simulink model "mpcfinal"  (R2022a)
settings: Solver=VariableStepAuto  StartTime=0.0  StopTime=100  RelTol=1e-3
libraries: mpclib x5
settings Model: Creator=Admin  LastModifiedBy=Admin

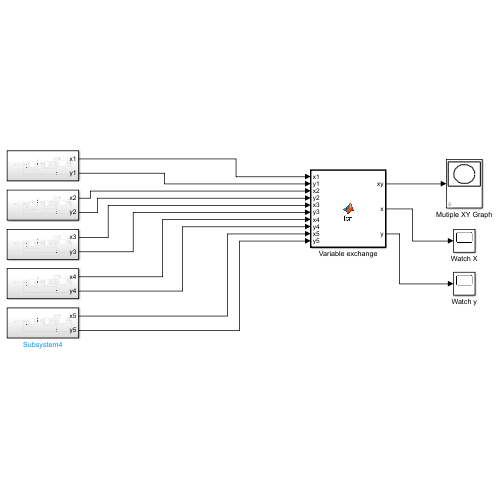
[thumbnail: Simulink's stored preview of the top-level diagram]
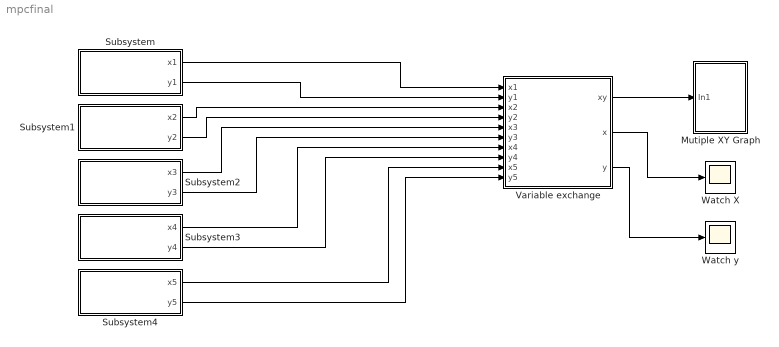
== system mpcfinal ==
  Mutiple XY Graph : Subsystem  mask(Mutiple XY Graph){number_of_trajectories=5, axis_limits=[-100 100 -100 100], sample_time=0.1}
      mask prompts: number_of_trajectories "Number of Trajectories"; axis_limits "Axis Limits"; sample_time "Sample Time"
      mask Display: plot([.05 .95 .95 .05 .05],[.45 .45 .95 .95 .45], 0.5+cos(0:0.1:2*pi)*0.3,0.7+sin(0:0.1:2*pi)*0.2)
  Subsystem : Subsystem
  Subsystem1 : Subsystem
  Subsystem2 : Subsystem
  Subsystem3 : Subsystem
  Subsystem4 : Subsystem
  Variable exchange : MATLAB Function  TreatAsAtomicUnit=on
  Watch X : Scope
  Watch y : Scope
  wires:
  Subsystem2/2(y3) -> Variable exchange/6(y3)
  Subsystem/2(y1) -> Variable exchange/2(y1)
  Subsystem4/2(y5) -> Variable exchange/10(y5)
  Subsystem2/1(x3) -> Variable exchange/5(x3)
  Subsystem4/1(x5) -> Variable exchange/9(x5)
  Variable exchange/1(xy) -> Mutiple XY Graph/1(In1)
  Variable exchange/2(x) -> Watch X/1
  Subsystem3/2(y4) -> Variable exchange/8(y4)
  Subsystem1/2(y2) -> Variable exchange/4(y2)
  Variable exchange/3(y) -> Watch y/1
  Subsystem1/1(x2) -> Variable exchange/3(x2)
  Subsystem/1(x1) -> Variable exchange/1(x1)
  Subsystem3/1(x4) -> Variable exchange/7(x4)

== system mpcfinal/Mutiple XY Graph ==
  In1 : Inport
  Level-2 MATLAB S-Function : M-S-Function  FunctionName=multiple_xy_graph  Parameters=number_of_trajectories,axis_limits
  Rate Transition : RateTransition  OutPortSampleTime=sample_time
  wires:
  In1/1 -> Rate Transition/1
  Rate Transition/1 -> Level-2 MATLAB S-Function/1

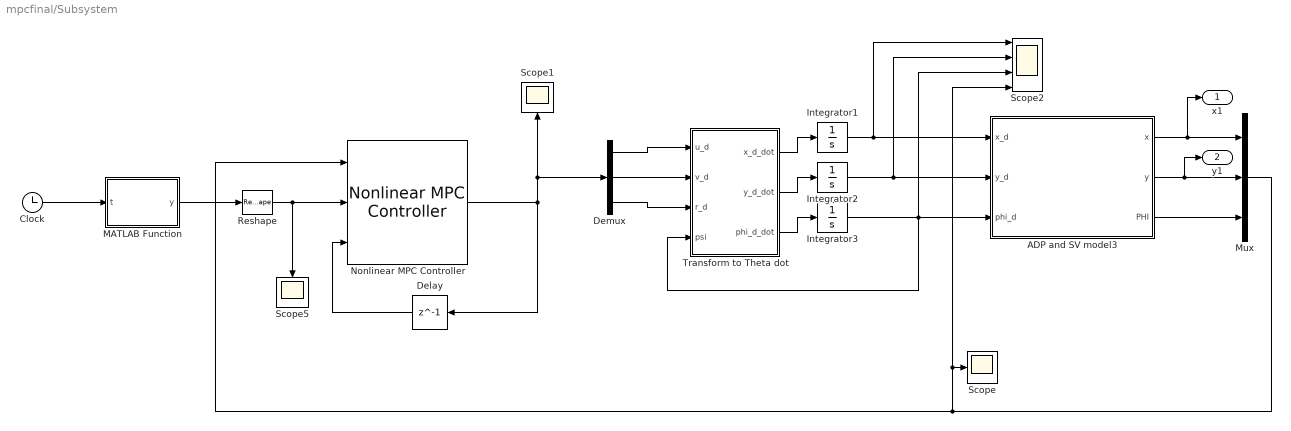
== system mpcfinal/Subsystem ==
  ADP and SV model3 : Subsystem
  Clock : Clock
  Delay : Delay  DelayLength=1
  Demux : Demux  Outputs=3
  Integrator1 : Integrator  InitialCondition=10
  Integrator2 : Integrator  InitialCondition=10
  Integrator3 : Integrator
  MATLAB Function : MATLAB Function  TreatAsAtomicUnit=on
  Mux : Mux  Inputs=3
  Nonlinear MPC Controller : mpclib/Nonlinear MPC Controller  nlmpcobj=nlobj  UseObjectTs=on  UseMEX=off  md_enabled=off  mvtarget_enabled=off  param_enabled=off  cost_enabled=off  mvseq_enabled=off  stateseq_enabled=off  ovseq_enabled=off  slack_enabled=off  status_enabled=off  ov_min=off  ov_max=off  mv_min=off  mv_max=off  mvrate_min=off  mvrate_max=off  state_min=off  state_max=off  ov_weight=off  mv_weight=off  mvrate_weight=off  ecr_weight=off  nlp_initialize=off
  Reshape : Reshape  OutputDimensionality=Customize  OutputDimensions=[1,3]
  Scope : Scope
  Scope1 : Scope
  Scope2 : Scope  NumInputPorts=4
  Scope5 : Scope
  Transform to Theta dot : MATLAB Function  TreatAsAtomicUnit=on
  x1 : Outport
  y1 : Outport  Port=2
  wires:
  Nonlinear MPC Controller/1 -> Demux/1, Scope1/1, Delay/1
  ADP and SV model3/2(y) -> y1/1, Mux/2
  ADP and SV model3/3(PHI) -> Mux/3
  Demux/1 -> Transform to Theta dot/1(u_d)
  Integrator2/1 -> ADP and SV model3/2(y_d), Scope2/2
  Clock/1 -> MATLAB Function/1(t)
  Transform to Theta dot/1(x_d_dot) -> Integrator1/1
  Reshape/1 -> Nonlinear MPC Controller/2, Scope5/1
  Integrator3/1 -> ADP and SV model3/3(phi_d), Transform to Theta dot/4(psi), Scope2/3
  MATLAB Function/1(y) -> Reshape/1
  Demux/3 -> Transform to Theta dot/3(r_d)
  ADP and SV model3/1(x) -> x1/1, Mux/1
  Delay/1 -> Nonlinear MPC Controller/3
  Transform to Theta dot/2(y_d_dot) -> Integrator2/1
  Demux/2 -> Transform to Theta dot/2(v_d)
  Mux/1 -> Scope2/4, Scope/1, Nonlinear MPC Controller/1
  Integrator1/1 -> Scope2/1, ADP and SV model3/1(x_d)
  Transform to Theta dot/3(phi_d_dot) -> Integrator3/1

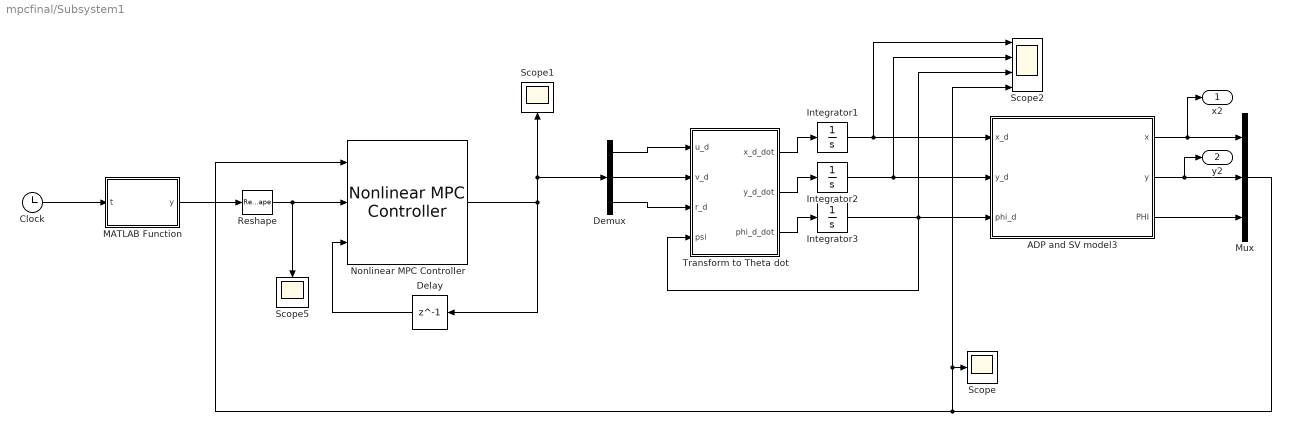
== system mpcfinal/Subsystem1 ==
  ADP and SV model3 : Subsystem
  Clock : Clock
  Delay : Delay  DelayLength=1
  Demux : Demux  Outputs=3
  Integrator1 : Integrator  InitialCondition=15
  Integrator2 : Integrator  InitialCondition=10
  Integrator3 : Integrator
  MATLAB Function : MATLAB Function  TreatAsAtomicUnit=on
  Mux : Mux  Inputs=3
  Nonlinear MPC Controller : mpclib/Nonlinear MPC Controller  nlmpcobj=nlobj  UseObjectTs=on  UseMEX=off  md_enabled=off  mvtarget_enabled=off  param_enabled=off  cost_enabled=off  mvseq_enabled=off  stateseq_enabled=off  ovseq_enabled=off  slack_enabled=off  status_enabled=off  ov_min=off  ov_max=off  mv_min=off  mv_max=off  mvrate_min=off  mvrate_max=off  state_min=off  state_max=off  ov_weight=off  mv_weight=off  mvrate_weight=off  ecr_weight=off  nlp_initialize=off
  Reshape : Reshape  OutputDimensionality=Customize  OutputDimensions=[1,3]
  Scope : Scope
  Scope1 : Scope
  Scope2 : Scope  NumInputPorts=4
  Scope5 : Scope
  Transform to Theta dot : MATLAB Function  TreatAsAtomicUnit=on
  x2 : Outport
  y2 : Outport  Port=2
  wires:
  Nonlinear MPC Controller/1 -> Demux/1, Scope1/1, Delay/1
  ADP and SV model3/2(y) -> y2/1, Mux/2
  ADP and SV model3/3(PHI) -> Mux/3
  Demux/1 -> Transform to Theta dot/1(u_d)
  Integrator2/1 -> ADP and SV model3/2(y_d), Scope2/2
  Clock/1 -> MATLAB Function/1(t)
  Transform to Theta dot/1(x_d_dot) -> Integrator1/1
  Reshape/1 -> Nonlinear MPC Controller/2, Scope5/1
  Integrator3/1 -> ADP and SV model3/3(phi_d), Transform to Theta dot/4(psi), Scope2/3
  MATLAB Function/1(y) -> Reshape/1
  Demux/3 -> Transform to Theta dot/3(r_d)
  ADP and SV model3/1(x) -> x2/1, Mux/1
  Delay/1 -> Nonlinear MPC Controller/3
  Transform to Theta dot/2(y_d_dot) -> Integrator2/1
  Demux/2 -> Transform to Theta dot/2(v_d)
  Mux/1 -> Scope2/4, Scope/1, Nonlinear MPC Controller/1
  Integrator1/1 -> Scope2/1, ADP and SV model3/1(x_d)
  Transform to Theta dot/3(phi_d_dot) -> Integrator3/1

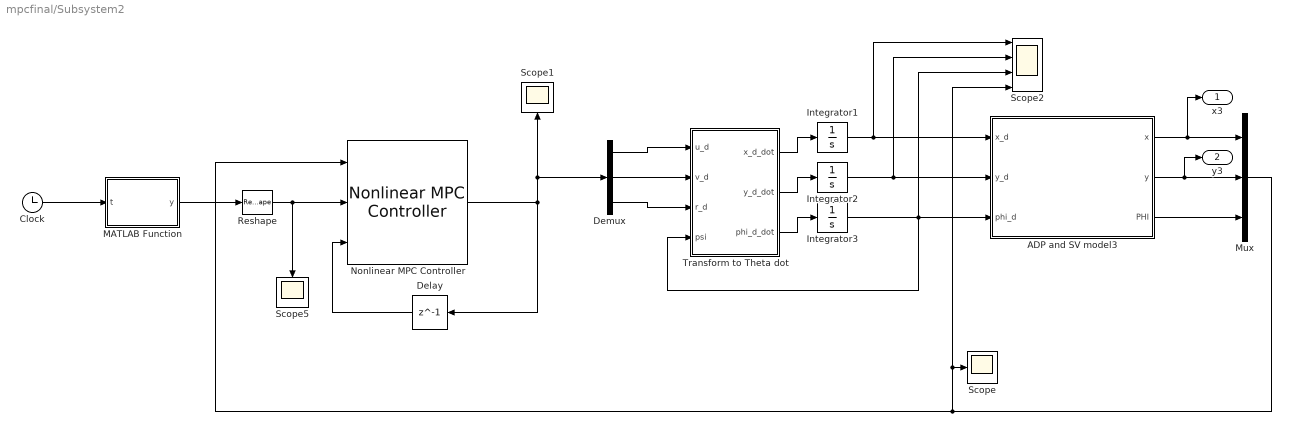
== system mpcfinal/Subsystem2 ==
  ADP and SV model3 : Subsystem
  Clock : Clock
  Delay : Delay  DelayLength=1
  Demux : Demux  Outputs=3
  Integrator1 : Integrator  InitialCondition=10
  Integrator2 : Integrator  InitialCondition=5
  Integrator3 : Integrator
  MATLAB Function : MATLAB Function  TreatAsAtomicUnit=on
  Mux : Mux  Inputs=3
  Nonlinear MPC Controller : mpclib/Nonlinear MPC Controller  nlmpcobj=nlobj  UseObjectTs=on  UseMEX=off  md_enabled=off  mvtarget_enabled=off  param_enabled=off  cost_enabled=off  mvseq_enabled=off  stateseq_enabled=off  ovseq_enabled=off  slack_enabled=off  status_enabled=off  ov_min=off  ov_max=off  mv_min=off  mv_max=off  mvrate_min=off  mvrate_max=off  state_min=off  state_max=off  ov_weight=off  mv_weight=off  mvrate_weight=off  ecr_weight=off  nlp_initialize=off
  Reshape : Reshape  OutputDimensionality=Customize  OutputDimensions=[1,3]
  Scope : Scope
  Scope1 : Scope
  Scope2 : Scope  NumInputPorts=4
  Scope5 : Scope
  Transform to Theta dot : MATLAB Function  TreatAsAtomicUnit=on
  x3 : Outport
  y3 : Outport  Port=2
  wires:
  Nonlinear MPC Controller/1 -> Demux/1, Scope1/1, Delay/1
  ADP and SV model3/2(y) -> y3/1, Mux/2
  ADP and SV model3/3(PHI) -> Mux/3
  Demux/1 -> Transform to Theta dot/1(u_d)
  Integrator2/1 -> ADP and SV model3/2(y_d), Scope2/2
  Clock/1 -> MATLAB Function/1(t)
  Transform to Theta dot/1(x_d_dot) -> Integrator1/1
  Reshape/1 -> Nonlinear MPC Controller/2, Scope5/1
  Integrator3/1 -> ADP and SV model3/3(phi_d), Transform to Theta dot/4(psi), Scope2/3
  MATLAB Function/1(y) -> Reshape/1
  Demux/3 -> Transform to Theta dot/3(r_d)
  ADP and SV model3/1(x) -> x3/1, Mux/1
  Delay/1 -> Nonlinear MPC Controller/3
  Transform to Theta dot/2(y_d_dot) -> Integrator2/1
  Demux/2 -> Transform to Theta dot/2(v_d)
  Mux/1 -> Scope2/4, Scope/1, Nonlinear MPC Controller/1
  Integrator1/1 -> Scope2/1, ADP and SV model3/1(x_d)
  Transform to Theta dot/3(phi_d_dot) -> Integrator3/1

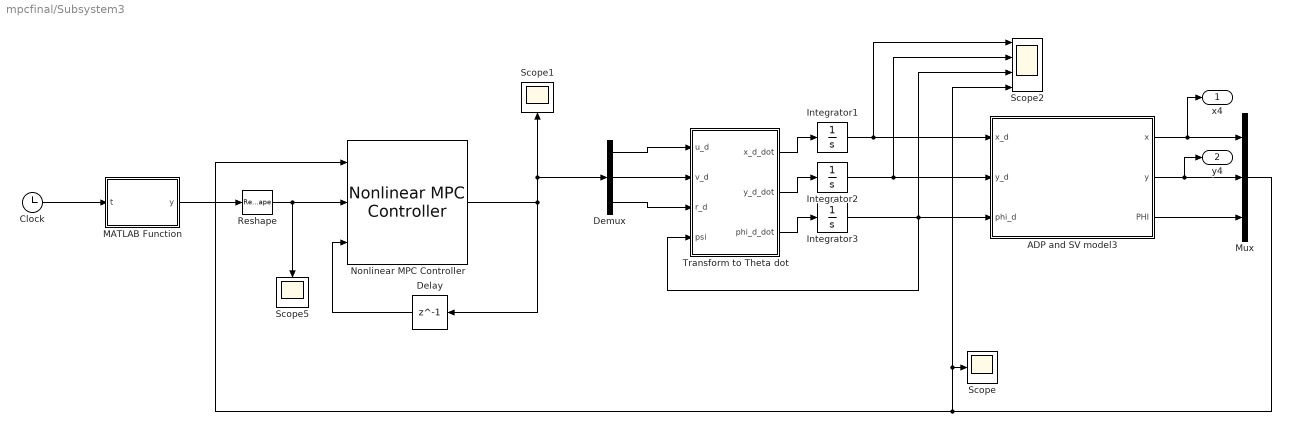
== system mpcfinal/Subsystem3 ==
  ADP and SV model3 : Subsystem
  Clock : Clock
  Delay : Delay  DelayLength=1
  Demux : Demux  Outputs=3
  Integrator1 : Integrator  InitialCondition=5
  Integrator2 : Integrator  InitialCondition=10
  Integrator3 : Integrator
  MATLAB Function : MATLAB Function  TreatAsAtomicUnit=on
  Mux : Mux  Inputs=3
  Nonlinear MPC Controller : mpclib/Nonlinear MPC Controller  nlmpcobj=nlobj  UseObjectTs=on  UseMEX=off  md_enabled=off  mvtarget_enabled=off  param_enabled=off  cost_enabled=off  mvseq_enabled=off  stateseq_enabled=off  ovseq_enabled=off  slack_enabled=off  status_enabled=off  ov_min=off  ov_max=off  mv_min=off  mv_max=off  mvrate_min=off  mvrate_max=off  state_min=off  state_max=off  ov_weight=off  mv_weight=off  mvrate_weight=off  ecr_weight=off  nlp_initialize=off
  Reshape : Reshape  OutputDimensionality=Customize  OutputDimensions=[1,3]
  Scope : Scope
  Scope1 : Scope
  Scope2 : Scope  NumInputPorts=4
  Scope5 : Scope
  Transform to Theta dot : MATLAB Function  TreatAsAtomicUnit=on
  x4 : Outport
  y4 : Outport  Port=2
  wires:
  Nonlinear MPC Controller/1 -> Demux/1, Scope1/1, Delay/1
  ADP and SV model3/2(y) -> y4/1, Mux/2
  ADP and SV model3/3(PHI) -> Mux/3
  Demux/1 -> Transform to Theta dot/1(u_d)
  Integrator2/1 -> ADP and SV model3/2(y_d), Scope2/2
  Clock/1 -> MATLAB Function/1(t)
  Transform to Theta dot/1(x_d_dot) -> Integrator1/1
  Reshape/1 -> Nonlinear MPC Controller/2, Scope5/1
  Integrator3/1 -> ADP and SV model3/3(phi_d), Transform to Theta dot/4(psi), Scope2/3
  MATLAB Function/1(y) -> Reshape/1
  Demux/3 -> Transform to Theta dot/3(r_d)
  ADP and SV model3/1(x) -> x4/1, Mux/1
  Delay/1 -> Nonlinear MPC Controller/3
  Transform to Theta dot/2(y_d_dot) -> Integrator2/1
  Demux/2 -> Transform to Theta dot/2(v_d)
  Mux/1 -> Scope2/4, Scope/1, Nonlinear MPC Controller/1
  Integrator1/1 -> Scope2/1, ADP and SV model3/1(x_d)
  Transform to Theta dot/3(phi_d_dot) -> Integrator3/1

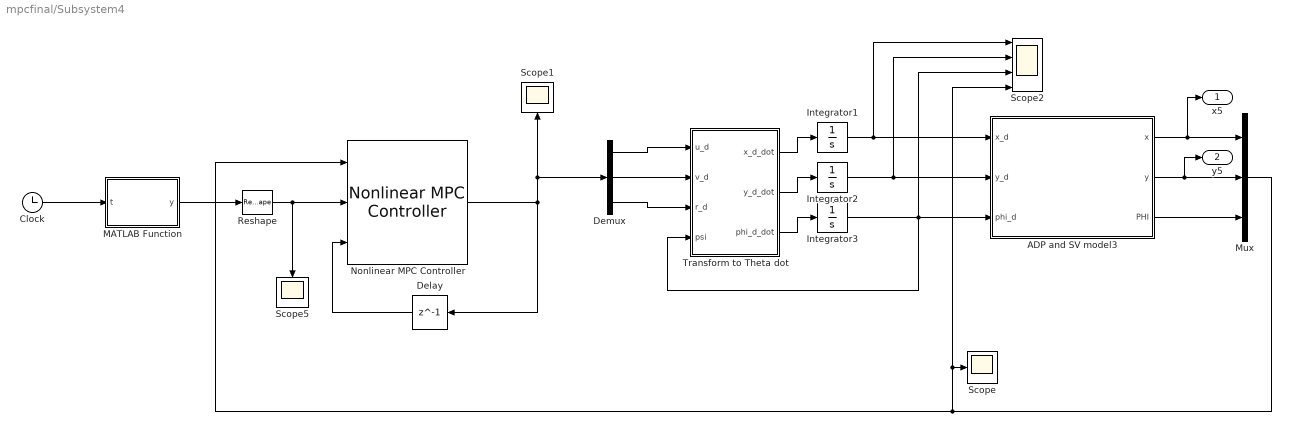
== system mpcfinal/Subsystem4 ==
  ADP and SV model3 : Subsystem
  Clock : Clock
  Delay : Delay  DelayLength=1
  Demux : Demux  Outputs=3
  Integrator1 : Integrator  InitialCondition=10
  Integrator2 : Integrator  InitialCondition=15
  Integrator3 : Integrator
  MATLAB Function : MATLAB Function  TreatAsAtomicUnit=on
  Mux : Mux  Inputs=3
  Nonlinear MPC Controller : mpclib/Nonlinear MPC Controller  nlmpcobj=nlobj  UseObjectTs=on  UseMEX=off  md_enabled=off  mvtarget_enabled=off  param_enabled=off  cost_enabled=off  mvseq_enabled=off  stateseq_enabled=off  ovseq_enabled=off  slack_enabled=off  status_enabled=off  ov_min=off  ov_max=off  mv_min=off  mv_max=off  mvrate_min=off  mvrate_max=off  state_min=off  state_max=off  ov_weight=off  mv_weight=off  mvrate_weight=off  ecr_weight=off  nlp_initialize=off
  Reshape : Reshape  OutputDimensionality=Customize  OutputDimensions=[1,3]
  Scope : Scope
  Scope1 : Scope
  Scope2 : Scope  NumInputPorts=4
  Scope5 : Scope
  Transform to Theta dot : MATLAB Function  TreatAsAtomicUnit=on
  x5 : Outport
  y5 : Outport  Port=2
  wires:
  Nonlinear MPC Controller/1 -> Demux/1, Scope1/1, Delay/1
  ADP and SV model3/2(y) -> y5/1, Mux/2
  ADP and SV model3/3(PHI) -> Mux/3
  Demux/1 -> Transform to Theta dot/1(u_d)
  Integrator2/1 -> ADP and SV model3/2(y_d), Scope2/2
  Clock/1 -> MATLAB Function/1(t)
  Transform to Theta dot/1(x_d_dot) -> Integrator1/1
  Reshape/1 -> Nonlinear MPC Controller/2, Scope5/1
  Integrator3/1 -> ADP and SV model3/3(phi_d), Transform to Theta dot/4(psi), Scope2/3
  MATLAB Function/1(y) -> Reshape/1
  Demux/3 -> Transform to Theta dot/3(r_d)
  ADP and SV model3/1(x) -> x5/1, Mux/1
  Delay/1 -> Nonlinear MPC Controller/3
  Transform to Theta dot/2(y_d_dot) -> Integrator2/1
  Demux/2 -> Transform to Theta dot/2(v_d)
  Mux/1 -> Scope2/4, Scope/1, Nonlinear MPC Controller/1
  Integrator1/1 -> Scope2/1, ADP and SV model3/1(x_d)
  Transform to Theta dot/3(phi_d_dot) -> Integrator3/1

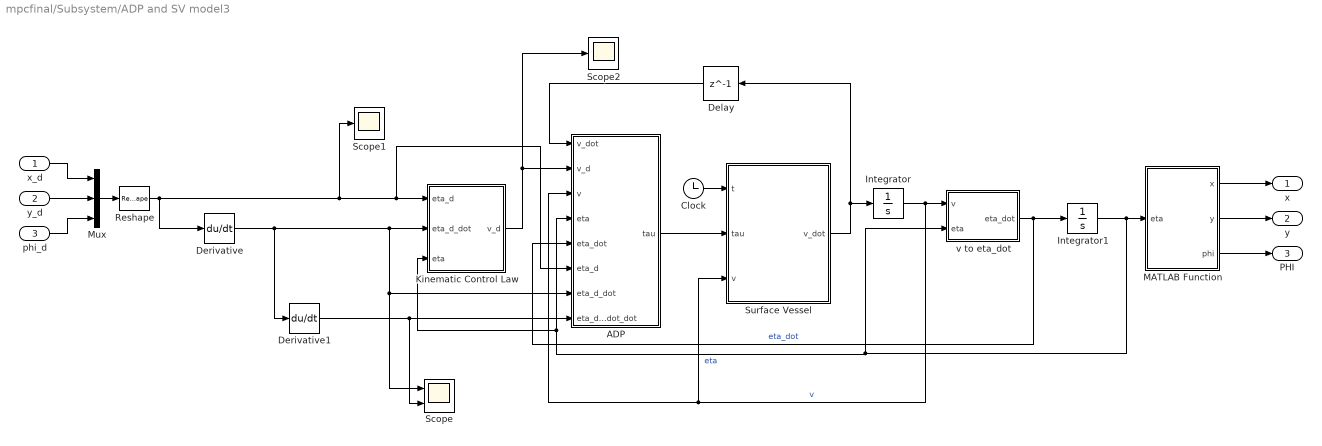
== system mpcfinal/Subsystem/ADP and SV model3 ==
  x_d : Inport
  y_d : Inport  Port=2
  phi_d : Inport  Port=3
  ADP : Subsystem
  Clock : Clock
  Delay : Delay  DelayLength=1  InitialCondition=[0;0;0]  SampleTime=1e-2
  Derivative : Derivative
  Derivative1 : Derivative
  Integrator : Integrator
  Integrator1 : Integrator  InitialCondition=[9;11;0.1]
  "Kinematic Control Law " : MATLAB Function  TreatAsAtomicUnit=on
  MATLAB Function : MATLAB Function  TreatAsAtomicUnit=on
  Mux : Mux  Inputs=3
  Reshape : Reshape  OutputDimensionality=Customize  OutputDimensions=[3,1]
  Scope : Scope  NumInputPorts=2
  Scope1 : Scope
  Scope2 : Scope
  "Surface Vessel " : MATLAB Function  TreatAsAtomicUnit=on
  v to eta_dot : MATLAB Function  TreatAsAtomicUnit=on
  x : Outport
  y : Outport  Port=2
  PHI : Outport  Port=3
  wires:
  x_d/1 -> Mux/1
  phi_d/1 -> Mux/3
  y_d/1 -> Mux/2
  Clock/1 -> "Surface Vessel "/1(t)
  "Surface Vessel "/1(v_dot) -> Delay/1, Integrator/1
  Integrator/1 -> ADP/3(v), "Surface Vessel "/3(v), v to eta_dot/1(v)  "v"
  Integrator1/1 -> ADP/4(eta), "Kinematic Control Law "/3(eta), v to eta_dot/2(eta), MATLAB Function/1(eta)  "eta"
  ADP/1(tau) -> "Surface Vessel "/2(tau)
  "Kinematic Control Law "/1(v_d) -> Scope2/1, ADP/2(v_d)
  Delay/1 -> ADP/1(v_dot)
  Reshape/1 -> Derivative/1, Scope1/1, ADP/6(eta_d), "Kinematic Control Law "/1(eta_d)
  v to eta_dot/1(eta_dot) -> ADP/5(eta_dot), Integrator1/1  "eta_dot"
  MATLAB Function/1(x) -> x/1
  MATLAB Function/2(y) -> y/1
  MATLAB Function/3(phi) -> PHI/1
  Mux/1 -> Reshape/1
  Derivative/1 -> Derivative1/1, ADP/7(eta_d_dot), Scope/1, "Kinematic Control Law "/2(eta_d_dot)
  Derivative1/1 -> Scope/2, ADP/8(eta_d_dot_dot)

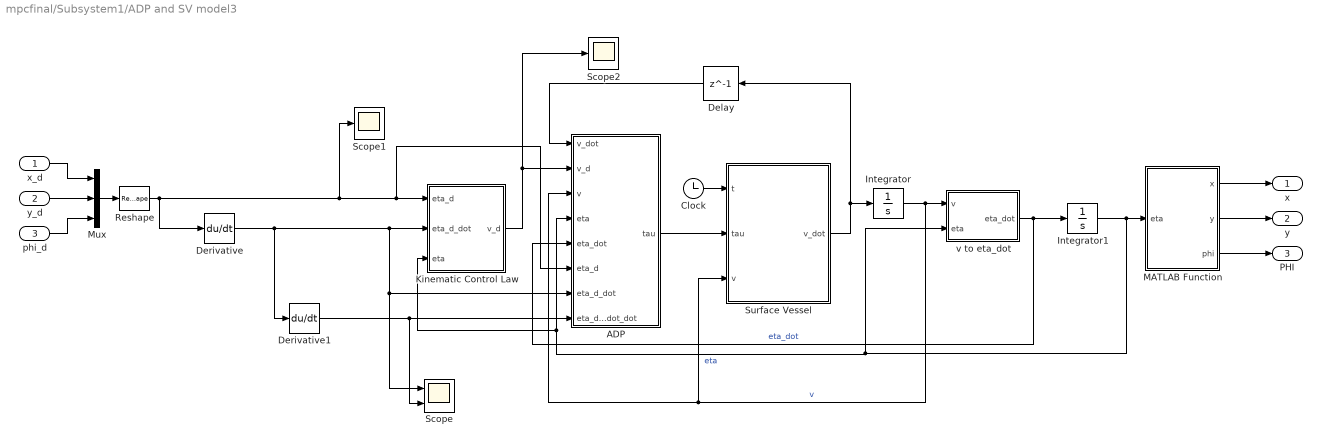
== system mpcfinal/Subsystem1/ADP and SV model3 ==
  x_d : Inport
  y_d : Inport  Port=2
  phi_d : Inport  Port=3
  ADP : Subsystem
  Clock : Clock
  Delay : Delay  DelayLength=1  InitialCondition=[0;0;0]  SampleTime=1e-2
  Derivative : Derivative
  Derivative1 : Derivative
  Integrator : Integrator
  Integrator1 : Integrator  InitialCondition=[14;11;0.1]
  "Kinematic Control Law " : MATLAB Function  TreatAsAtomicUnit=on
  MATLAB Function : MATLAB Function  TreatAsAtomicUnit=on
  Mux : Mux  Inputs=3
  Reshape : Reshape  OutputDimensionality=Customize  OutputDimensions=[3,1]
  Scope : Scope  NumInputPorts=2
  Scope1 : Scope
  Scope2 : Scope
  "Surface Vessel " : MATLAB Function  TreatAsAtomicUnit=on
  v to eta_dot : MATLAB Function  TreatAsAtomicUnit=on
  x : Outport
  y : Outport  Port=2
  PHI : Outport  Port=3
  wires:
  x_d/1 -> Mux/1
  phi_d/1 -> Mux/3
  y_d/1 -> Mux/2
  Clock/1 -> "Surface Vessel "/1(t)
  "Surface Vessel "/1(v_dot) -> Delay/1, Integrator/1
  Integrator/1 -> ADP/3(v), "Surface Vessel "/3(v), v to eta_dot/1(v)  "v"
  Integrator1/1 -> ADP/4(eta), "Kinematic Control Law "/3(eta), v to eta_dot/2(eta), MATLAB Function/1(eta)  "eta"
  ADP/1(tau) -> "Surface Vessel "/2(tau)
  "Kinematic Control Law "/1(v_d) -> Scope2/1, ADP/2(v_d)
  Delay/1 -> ADP/1(v_dot)
  Reshape/1 -> Derivative/1, Scope1/1, ADP/6(eta_d), "Kinematic Control Law "/1(eta_d)
  v to eta_dot/1(eta_dot) -> ADP/5(eta_dot), Integrator1/1  "eta_dot"
  MATLAB Function/1(x) -> x/1
  MATLAB Function/2(y) -> y/1
  MATLAB Function/3(phi) -> PHI/1
  Mux/1 -> Reshape/1
  Derivative/1 -> Derivative1/1, ADP/7(eta_d_dot), Scope/1, "Kinematic Control Law "/2(eta_d_dot)
  Derivative1/1 -> Scope/2, ADP/8(eta_d_dot_dot)

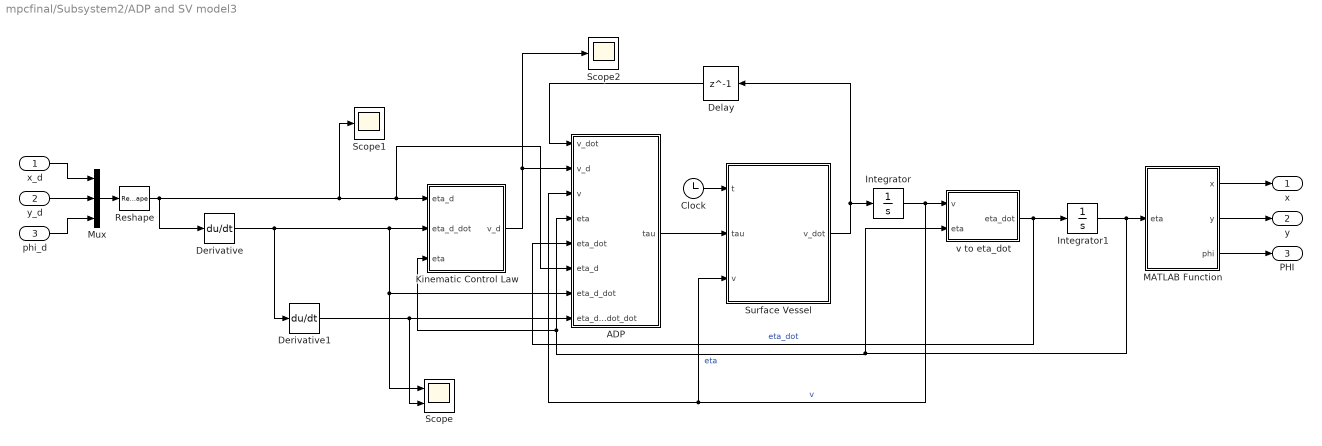
== system mpcfinal/Subsystem2/ADP and SV model3 ==
  x_d : Inport
  y_d : Inport  Port=2
  phi_d : Inport  Port=3
  ADP : Subsystem
  Clock : Clock
  Delay : Delay  DelayLength=1  InitialCondition=[0;0;0]  SampleTime=1e-2
  Derivative : Derivative
  Derivative1 : Derivative
  Integrator : Integrator
  Integrator1 : Integrator  InitialCondition=[9;5;-0.1]
  "Kinematic Control Law " : MATLAB Function  TreatAsAtomicUnit=on
  MATLAB Function : MATLAB Function  TreatAsAtomicUnit=on
  Mux : Mux  Inputs=3
  Reshape : Reshape  OutputDimensionality=Customize  OutputDimensions=[3,1]
  Scope : Scope  NumInputPorts=2
  Scope1 : Scope
  Scope2 : Scope
  "Surface Vessel " : MATLAB Function  TreatAsAtomicUnit=on
  v to eta_dot : MATLAB Function  TreatAsAtomicUnit=on
  x : Outport
  y : Outport  Port=2
  PHI : Outport  Port=3
  wires:
  x_d/1 -> Mux/1
  phi_d/1 -> Mux/3
  y_d/1 -> Mux/2
  Clock/1 -> "Surface Vessel "/1(t)
  "Surface Vessel "/1(v_dot) -> Delay/1, Integrator/1
  Integrator/1 -> ADP/3(v), "Surface Vessel "/3(v), v to eta_dot/1(v)  "v"
  Integrator1/1 -> ADP/4(eta), "Kinematic Control Law "/3(eta), v to eta_dot/2(eta), MATLAB Function/1(eta)  "eta"
  ADP/1(tau) -> "Surface Vessel "/2(tau)
  "Kinematic Control Law "/1(v_d) -> Scope2/1, ADP/2(v_d)
  Delay/1 -> ADP/1(v_dot)
  Reshape/1 -> Derivative/1, Scope1/1, ADP/6(eta_d), "Kinematic Control Law "/1(eta_d)
  v to eta_dot/1(eta_dot) -> ADP/5(eta_dot), Integrator1/1  "eta_dot"
  MATLAB Function/1(x) -> x/1
  MATLAB Function/2(y) -> y/1
  MATLAB Function/3(phi) -> PHI/1
  Mux/1 -> Reshape/1
  Derivative/1 -> Derivative1/1, ADP/7(eta_d_dot), Scope/1, "Kinematic Control Law "/2(eta_d_dot)
  Derivative1/1 -> Scope/2, ADP/8(eta_d_dot_dot)

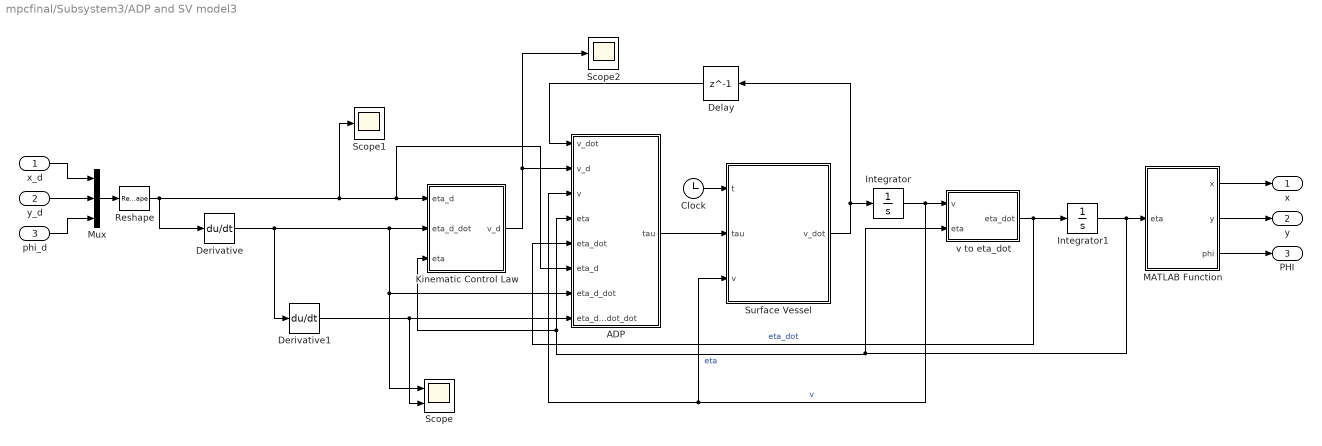
== system mpcfinal/Subsystem3/ADP and SV model3 ==
  x_d : Inport
  y_d : Inport  Port=2
  phi_d : Inport  Port=3
  ADP : Subsystem
  Clock : Clock
  Delay : Delay  DelayLength=1  InitialCondition=[0;0;0]  SampleTime=1e-2
  Derivative : Derivative
  Derivative1 : Derivative
  Integrator : Integrator
  Integrator1 : Integrator  InitialCondition=[6;11;0.1]
  "Kinematic Control Law " : MATLAB Function  TreatAsAtomicUnit=on
  MATLAB Function : MATLAB Function  TreatAsAtomicUnit=on
  Mux : Mux  Inputs=3
  Reshape : Reshape  OutputDimensionality=Customize  OutputDimensions=[3,1]
  Scope : Scope  NumInputPorts=2
  Scope1 : Scope
  Scope2 : Scope
  "Surface Vessel " : MATLAB Function  TreatAsAtomicUnit=on
  v to eta_dot : MATLAB Function  TreatAsAtomicUnit=on
  x : Outport
  y : Outport  Port=2
  PHI : Outport  Port=3
  wires:
  x_d/1 -> Mux/1
  phi_d/1 -> Mux/3
  y_d/1 -> Mux/2
  Clock/1 -> "Surface Vessel "/1(t)
  "Surface Vessel "/1(v_dot) -> Delay/1, Integrator/1
  Integrator/1 -> ADP/3(v), "Surface Vessel "/3(v), v to eta_dot/1(v)  "v"
  Integrator1/1 -> ADP/4(eta), "Kinematic Control Law "/3(eta), v to eta_dot/2(eta), MATLAB Function/1(eta)  "eta"
  ADP/1(tau) -> "Surface Vessel "/2(tau)
  "Kinematic Control Law "/1(v_d) -> Scope2/1, ADP/2(v_d)
  Delay/1 -> ADP/1(v_dot)
  Reshape/1 -> Derivative/1, Scope1/1, ADP/6(eta_d), "Kinematic Control Law "/1(eta_d)
  v to eta_dot/1(eta_dot) -> ADP/5(eta_dot), Integrator1/1  "eta_dot"
  MATLAB Function/1(x) -> x/1
  MATLAB Function/2(y) -> y/1
  MATLAB Function/3(phi) -> PHI/1
  Mux/1 -> Reshape/1
  Derivative/1 -> Derivative1/1, ADP/7(eta_d_dot), Scope/1, "Kinematic Control Law "/2(eta_d_dot)
  Derivative1/1 -> Scope/2, ADP/8(eta_d_dot_dot)

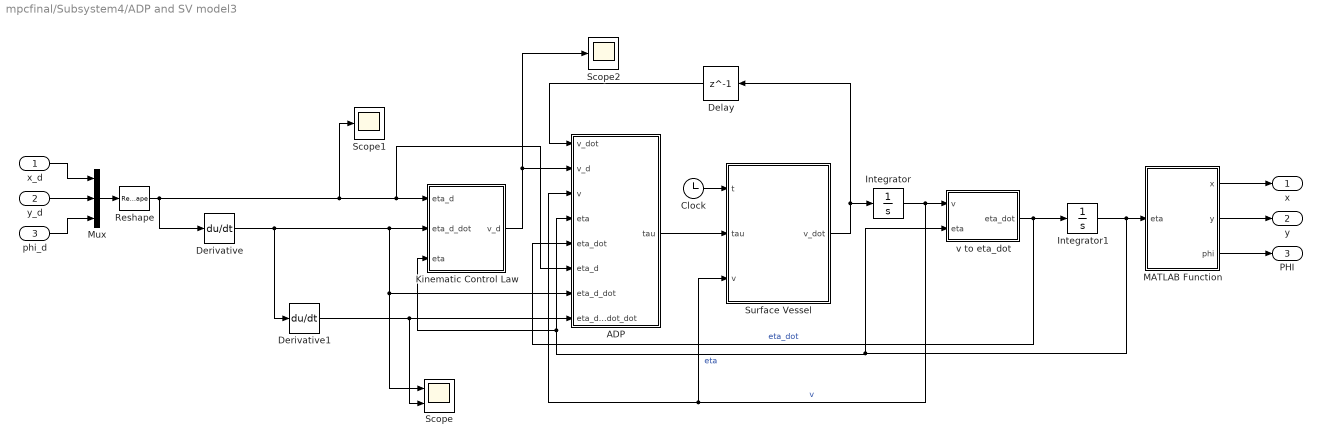
== system mpcfinal/Subsystem4/ADP and SV model3 ==
  x_d : Inport
  y_d : Inport  Port=2
  phi_d : Inport  Port=3
  ADP : Subsystem
  Clock : Clock
  Delay : Delay  DelayLength=1  InitialCondition=[0;0;0]  SampleTime=1e-2
  Derivative : Derivative
  Derivative1 : Derivative
  Integrator : Integrator
  Integrator1 : Integrator  InitialCondition=[9;14;-0.1]
  "Kinematic Control Law " : MATLAB Function  TreatAsAtomicUnit=on
  MATLAB Function : MATLAB Function  TreatAsAtomicUnit=on
  Mux : Mux  Inputs=3
  Reshape : Reshape  OutputDimensionality=Customize  OutputDimensions=[3,1]
  Scope : Scope  NumInputPorts=2
  Scope1 : Scope
  Scope2 : Scope
  "Surface Vessel " : MATLAB Function  TreatAsAtomicUnit=on
  v to eta_dot : MATLAB Function  TreatAsAtomicUnit=on
  x : Outport
  y : Outport  Port=2
  PHI : Outport  Port=3
  wires:
  x_d/1 -> Mux/1
  phi_d/1 -> Mux/3
  y_d/1 -> Mux/2
  Clock/1 -> "Surface Vessel "/1(t)
  "Surface Vessel "/1(v_dot) -> Delay/1, Integrator/1
  Integrator/1 -> ADP/3(v), "Surface Vessel "/3(v), v to eta_dot/1(v)  "v"
  Integrator1/1 -> ADP/4(eta), "Kinematic Control Law "/3(eta), v to eta_dot/2(eta), MATLAB Function/1(eta)  "eta"
  ADP/1(tau) -> "Surface Vessel "/2(tau)
  "Kinematic Control Law "/1(v_d) -> Scope2/1, ADP/2(v_d)
  Delay/1 -> ADP/1(v_dot)
  Reshape/1 -> Derivative/1, Scope1/1, ADP/6(eta_d), "Kinematic Control Law "/1(eta_d)
  v to eta_dot/1(eta_dot) -> ADP/5(eta_dot), Integrator1/1  "eta_dot"
  MATLAB Function/1(x) -> x/1
  MATLAB Function/2(y) -> y/1
  MATLAB Function/3(phi) -> PHI/1
  Mux/1 -> Reshape/1
  Derivative/1 -> Derivative1/1, ADP/7(eta_d_dot), Scope/1, "Kinematic Control Law "/2(eta_d_dot)
  Derivative1/1 -> Scope/2, ADP/8(eta_d_dot_dot)

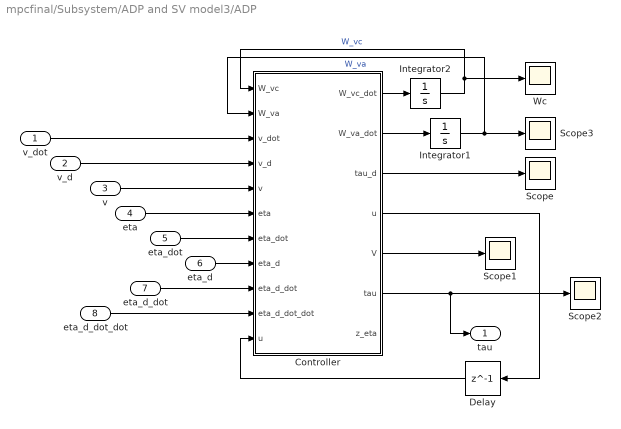
== system mpcfinal/Subsystem/ADP and SV model3/ADP ==
  v_dot : Inport
  v_d : Inport  Port=2
  v : Inport  Port=3
  eta : Inport  Port=4
  eta_dot : Inport  Port=5
  eta_d : Inport  Port=6
  eta_d_dot : Inport  Port=7
  eta_d_dot_dot : Inport  Port=8
  Controller : MATLAB Function  TreatAsAtomicUnit=on
  Delay : Delay  DelayLength=1  InitialCondition=[0;0;0]  SampleTime=1e-2
  Integrator1 : Integrator  InitialCondition=zeros(12,1)+0.1
  Integrator2 : Integrator  InitialCondition=zeros(12,1)
  Scope{,1..3} (4 alike) : Scope
  Wc : Scope
  tau : Outport
  wires:
  Controller/1(W_vc_dot) -> Integrator2/1
  Controller/2(W_va_dot) -> Integrator1/1
  Integrator1/1 -> Scope3/1, Controller/2(W_va)  "W_va"
  Integrator2/1 -> Controller/1(W_vc), Wc/1  "W_vc"
  v_d/1 -> Controller/4(v_d)
  v/1 -> Controller/5(v)
  eta/1 -> Controller/6(eta)
  eta_d/1 -> Controller/8(eta_d)
  eta_d_dot/1 -> Controller/9(eta_d_dot)
  eta_d_dot_dot/1 -> Controller/10(eta_d_dot_dot)
  eta_dot/1 -> Controller/7(eta_dot)
  Delay/1 -> Controller/11("u ")
  v_dot/1 -> Controller/3(v_dot)
  Controller/4(u) -> Delay/1
  Controller/6(tau) -> tau/1, Scope2/1
  Controller/3(tau_d) -> Scope/1
  Controller/5(V) -> Scope1/1

== system mpcfinal/Subsystem1/ADP and SV model3/ADP ==
  v_dot : Inport
  v_d : Inport  Port=2
  v : Inport  Port=3
  eta : Inport  Port=4
  eta_dot : Inport  Port=5
  eta_d : Inport  Port=6
  eta_d_dot : Inport  Port=7
  eta_d_dot_dot : Inport  Port=8
  Controller : MATLAB Function  TreatAsAtomicUnit=on
  Delay : Delay  DelayLength=1  InitialCondition=[0;0;0]  SampleTime=1e-2
  Integrator1 : Integrator  InitialCondition=zeros(12,1)+0.1
  Integrator2 : Integrator  InitialCondition=zeros(12,1)
  Scope{,1..3} (4 alike) : Scope
  Wc : Scope
  tau : Outport
  wires:
  Controller/1(W_vc_dot) -> Integrator2/1
  Controller/2(W_va_dot) -> Integrator1/1
  Integrator1/1 -> Scope3/1, Controller/2(W_va)  "W_va"
  Integrator2/1 -> Controller/1(W_vc), Wc/1  "W_vc"
  v_d/1 -> Controller/4(v_d)
  v/1 -> Controller/5(v)
  eta/1 -> Controller/6(eta)
  eta_d/1 -> Controller/8(eta_d)
  eta_d_dot/1 -> Controller/9(eta_d_dot)
  eta_d_dot_dot/1 -> Controller/10(eta_d_dot_dot)
  eta_dot/1 -> Controller/7(eta_dot)
  Delay/1 -> Controller/11("u ")
  v_dot/1 -> Controller/3(v_dot)
  Controller/4(u) -> Delay/1
  Controller/6(tau) -> tau/1, Scope2/1
  Controller/3(tau_d) -> Scope/1
  Controller/5(V) -> Scope1/1

== system mpcfinal/Subsystem2/ADP and SV model3/ADP ==
  v_dot : Inport
  v_d : Inport  Port=2
  v : Inport  Port=3
  eta : Inport  Port=4
  eta_dot : Inport  Port=5
  eta_d : Inport  Port=6
  eta_d_dot : Inport  Port=7
  eta_d_dot_dot : Inport  Port=8
  Controller : MATLAB Function  TreatAsAtomicUnit=on
  Delay : Delay  DelayLength=1  InitialCondition=[0;0;0]  SampleTime=1e-2
  Integrator1 : Integrator  InitialCondition=zeros(12,1)+0.1
  Integrator2 : Integrator  InitialCondition=zeros(12,1)
  Scope{,1..3} (4 alike) : Scope
  Wc : Scope
  tau : Outport
  wires:
  Controller/1(W_vc_dot) -> Integrator2/1
  Controller/2(W_va_dot) -> Integrator1/1
  Integrator1/1 -> Scope3/1, Controller/2(W_va)  "W_va"
  Integrator2/1 -> Controller/1(W_vc), Wc/1  "W_vc"
  v_d/1 -> Controller/4(v_d)
  v/1 -> Controller/5(v)
  eta/1 -> Controller/6(eta)
  eta_d/1 -> Controller/8(eta_d)
  eta_d_dot/1 -> Controller/9(eta_d_dot)
  eta_d_dot_dot/1 -> Controller/10(eta_d_dot_dot)
  eta_dot/1 -> Controller/7(eta_dot)
  Delay/1 -> Controller/11("u ")
  v_dot/1 -> Controller/3(v_dot)
  Controller/4(u) -> Delay/1
  Controller/6(tau) -> tau/1, Scope2/1
  Controller/3(tau_d) -> Scope/1
  Controller/5(V) -> Scope1/1

== system mpcfinal/Subsystem3/ADP and SV model3/ADP ==
  v_dot : Inport
  v_d : Inport  Port=2
  v : Inport  Port=3
  eta : Inport  Port=4
  eta_dot : Inport  Port=5
  eta_d : Inport  Port=6
  eta_d_dot : Inport  Port=7
  eta_d_dot_dot : Inport  Port=8
  Controller : MATLAB Function  TreatAsAtomicUnit=on
  Delay : Delay  DelayLength=1  InitialCondition=[0;0;0]  SampleTime=1e-2
  Integrator1 : Integrator  InitialCondition=zeros(12,1)+0.1
  Integrator2 : Integrator  InitialCondition=zeros(12,1)
  Scope{,1..3} (4 alike) : Scope
  Wc : Scope
  tau : Outport
  wires:
  Controller/1(W_vc_dot) -> Integrator2/1
  Controller/2(W_va_dot) -> Integrator1/1
  Integrator1/1 -> Scope3/1, Controller/2(W_va)  "W_va"
  Integrator2/1 -> Controller/1(W_vc), Wc/1  "W_vc"
  v_d/1 -> Controller/4(v_d)
  v/1 -> Controller/5(v)
  eta/1 -> Controller/6(eta)
  eta_d/1 -> Controller/8(eta_d)
  eta_d_dot/1 -> Controller/9(eta_d_dot)
  eta_d_dot_dot/1 -> Controller/10(eta_d_dot_dot)
  eta_dot/1 -> Controller/7(eta_dot)
  Delay/1 -> Controller/11("u ")
  v_dot/1 -> Controller/3(v_dot)
  Controller/4(u) -> Delay/1
  Controller/6(tau) -> tau/1, Scope2/1
  Controller/3(tau_d) -> Scope/1
  Controller/5(V) -> Scope1/1

== system mpcfinal/Subsystem4/ADP and SV model3/ADP ==
  v_dot : Inport
  v_d : Inport  Port=2
  v : Inport  Port=3
  eta : Inport  Port=4
  eta_dot : Inport  Port=5
  eta_d : Inport  Port=6
  eta_d_dot : Inport  Port=7
  eta_d_dot_dot : Inport  Port=8
  Controller : MATLAB Function  TreatAsAtomicUnit=on
  Delay : Delay  DelayLength=1  InitialCondition=[0;0;0]  SampleTime=1e-2
  Integrator1 : Integrator  InitialCondition=zeros(12,1)+0.1
  Integrator2 : Integrator  InitialCondition=zeros(12,1)
  Scope{,1..3} (4 alike) : Scope
  Wc : Scope
  tau : Outport
  wires:
  Controller/1(W_vc_dot) -> Integrator2/1
  Controller/2(W_va_dot) -> Integrator1/1
  Integrator1/1 -> Scope3/1, Controller/2(W_va)  "W_va"
  Integrator2/1 -> Controller/1(W_vc), Wc/1  "W_vc"
  v_d/1 -> Controller/4(v_d)
  v/1 -> Controller/5(v)
  eta/1 -> Controller/6(eta)
  eta_d/1 -> Controller/8(eta_d)
  eta_d_dot/1 -> Controller/9(eta_d_dot)
  eta_d_dot_dot/1 -> Controller/10(eta_d_dot_dot)
  eta_dot/1 -> Controller/7(eta_dot)
  Delay/1 -> Controller/11("u ")
  v_dot/1 -> Controller/3(v_dot)
  Controller/4(u) -> Delay/1
  Controller/6(tau) -> tau/1, Scope2/1
  Controller/3(tau_d) -> Scope/1
  Controller/5(V) -> Scope1/1

== matlab function mpcfinal/Subsystem1/Transform to Theta dot ==
  data: u_d input; x_d_dot output; v_d input; r_d input; y_d_dot output; phi_d_dot output; psi input
function [x_d_dot,y_d_dot,phi_d_dot] = fcn(u_d,v_d,r_d,psi)
    x_d_dot = u_d*cos(psi) - v_d*sin(psi);
    y_d_dot = u_d*sin(psi) + v_d*cos(psi);
    phi_d_dot = r_d;

== matlab function mpcfinal/Subsystem2/ADP and SV model3/ADP/Controller ==
  data: W_vc input; W_vc_dot output; W_va_dot output; tau_d output; W_va input; v_dot input; v_d input; v input; eta input; eta_dot input; eta_d input; eta_d_dot input; eta_d_dot_dot input; u input; u output; V output; tau output; z_eta output
 function [W_vc_dot, W_va_dot, tau_d, u, V, tau, z_eta] = fcn(W_vc, W_va, v_dot, v_d, v,...
    eta, eta_dot, eta_d, eta_d_dot, eta_d_dot_dot,u)
M = [28.135,0,0;0,45.568,0;0,0,131.423];
C = [0,0,-45.568*v(2);0,0,28.135*v(1);-8.7165*v(2),-8.7165*v(1),0];
D = [100,0,0;0,200,0;0,0,150];
invM = inv(M);
beta_eta = 0.3;
eta_c = 10;
eta_a1 = 10;
eta_a2 = 20;
nuy = 0.01;
GAMMA = 20; %%khong cap nhat
%%
z_eta = eta-eta_d;
z_v = v - v_d;
x = [z_v;z_eta;eta_d];
z_eta_dot = eta_dot - eta_d_dot;

gradPhi = [2*x(1),0,0;...
             x(2),x(1),0;...
             x(3),0,x(1);...
             0,2*x(2),0;...
             0,x(3),x(2);...
             0,0,2*x(3);...
              2*x(1)*x(7)^2,0,0;...
              0,2*x(2)*x(8)^2,0;...
              0,0,2*x(3)*x(9)^2;...
              2*x(1)*x(4)^2,0,0;...
              0,2*x(2)*x(5)^2,0;...
              0,0,2*x(3)*x(6)^2]; 
          %size 12x3
Phi = [x(1)^2; x(1)*x(2); x(1)*x(3); x(2)^2; x(2)*x(3); x(3)^2; x(1)^2*x(7)^2; x(2)^2*x(8)^2; ...
    x(3)^2*x(9)^2; x(1)^2*x(4)^2; x(2)^2*x(5)^2; x(3)^2*x(6)^2];
V = W_vc'*Phi;    
J = [cos(eta(3)),-sin(eta(3)),0;sin(eta(3)),cos(eta(3)),0;0,0,1];

J_dot = [-sin(eta(3))*v(3), -cos(eta(3))*v(3), 0;
      cos(eta(3))*v(3), -sin(eta(3))*v(3), 0;
             0, 0, 0];
         

%%
v_d_dot = J_dot'*(eta_d_dot-beta_eta*z_eta)+J'*(eta_d_dot_dot-beta_eta*z_eta_dot);
delta_hjb = W_vc'*gradPhi*(v_dot-v_d_dot)+z_v'*z_v+u'*u;
omega = gradPhi*(v_dot-v_d_dot);    %size 12x1

W_vc_dot = -eta_c*GAMMA*omega/(1+nuy*(omega'*GAMMA*omega))*delta_hjb;
W_va_dot = -eta_a1/sqrt(1+omega'*omega)*gradPhi*(invM*invM')*gradPhi'*(W_va-W_vc)*delta_hjb...
-eta_a2*(W_va - W_vc);

tau_d = M*v_d_dot+C*v_d+D*v_d;

u = -1/2*invM'*gradPhi'*W_va;



tau = tau_d + u;
 end

== matlab function mpcfinal/Subsystem2/ADP and SV model3/Kinematic Control Law  ==
  data: eta_d input; v_d output; eta_d_dot input; eta input
function v_d = fcn(eta_d,eta_d_dot, eta)
beta_eta = 0.3;

J = [cos(eta(3)),-sin(eta(3)),0;sin(eta(3)),cos(eta(3)),0;0,0,1];
z_eta = eta - eta_d;
v_d = J'*(eta_d_dot-beta_eta*z_eta);
end

== matlab function mpcfinal/Subsystem2/ADP and SV model3/MATLAB Function ==
  data: x output; eta input; y output; phi output
function [x,y,phi] = fcn(eta)
x = eta(1);
y = eta(2);
phi = eta(3);

== matlab function mpcfinal/Subsystem2/ADP and SV model3/Surface Vessel  ==
  settings: updateMethod=DISCRETE
  data: t input; tau input; v_dot output; v input
function v_dot  = fcn(t, tau,v)
%%

M = [28.135,0,0;0,45.568,0;0,0,131.423];
C = [0,0,-45.568*v(2);0,0,28.135*v(1);-8.7165*v(2),-8.7165*v(1),0];
D = [100,0,0;0,200,0;0,0,150];
 
invM = inv(M);

%%
if (t < 15)
    flag = 1;
else 
    flag = 0;
end
noise = zeros(3,1);
% noise(1) = (50*sin(25*t) + 65*sin(45*(t-1)) + 45*sin(20*(t-0.5)) + 55*sin(35*(t-1.5)))*flag;
% noise(2) = (20*sin(25*t) + 10*sin(45*(t-1)) + 16*sin(20*(t-0.5)) + 20*sin(35*(t-1.5)))*flag;
% noise(3) = (9*sin(25*t) + 10*sin(45*(t-1)) + 14*sin(20*(t-0.5)) + 30*sin(35*(t-1.5)))*flag;

noise(1) = (10*sin(25*t) + 16*sin(45*(t-1)) + 15*sin(20*(t-0.5)) + 10*sin(35*(t-1.5)))*flag;
noise(2) = (50*sin(25*t) + 50*sin(45*(t-1)) + 40*sin(20*(t-0.5)) + 50*sin(35*(t-1.5)))*flag;
noise(3) = (40*sin(25*t) + 30*sin(45*(t-1)) + 45*sin(20*(t-0.5)) + 40*sin(35*(t-1.5)))*flag;

v_dot = -invM*C*v-invM*D*v+invM*(tau + noise);

== matlab function mpcfinal/Subsystem2/ADP and SV model3/v to eta_dot ==
  data: v input; eta_dot output; eta input
function eta_dot = fcn(v,eta)
J = [cos(eta(3)),-sin(eta(3)),0;sin(eta(3)),cos(eta(3)),0;0,0,1];
eta_dot = J*v;

== matlab function mpcfinal/Subsystem2/MATLAB Function ==
  data: t input; y output
function y = fcn(t)

y = [10+0.5*t+5*sin(0.05*t),5+0.5*t,0];
end

== matlab function mpcfinal/Subsystem2/Transform to Theta dot ==
  data: u_d input; x_d_dot output; v_d input; r_d input; y_d_dot output; phi_d_dot output; psi input
function [x_d_dot,y_d_dot,phi_d_dot] = fcn(u_d,v_d,r_d,psi)
    x_d_dot = u_d*cos(psi) - v_d*sin(psi);
    y_d_dot = u_d*sin(psi) + v_d*cos(psi);
    phi_d_dot = r_d;

== matlab function mpcfinal/Subsystem3/ADP and SV model3/ADP/Controller ==
  data: W_vc input; W_vc_dot output; W_va_dot output; tau_d output; W_va input; v_dot input; v_d input; v input; eta input; eta_dot input; eta_d input; eta_d_dot input; eta_d_dot_dot input; u input; u output; V output; tau output; z_eta output
 function [W_vc_dot, W_va_dot, tau_d, u, V, tau, z_eta] = fcn(W_vc, W_va, v_dot, v_d, v,...
    eta, eta_dot, eta_d, eta_d_dot, eta_d_dot_dot,u)
M = [28.135,0,0;0,45.568,0;0,0,131.423];
C = [0,0,-45.568*v(2);0,0,28.135*v(1);-8.7165*v(2),-8.7165*v(1),0];
D = [100,0,0;0,200,0;0,0,150];
invM = inv(M);
beta_eta = 0.3;
eta_c = 10;
eta_a1 = 10;
eta_a2 = 20;
nuy = 0.01;
GAMMA = 20; %%khong cap nhat
%%
z_eta = eta-eta_d;
z_v = v - v_d;
x = [z_v;z_eta;eta_d];
z_eta_dot = eta_dot - eta_d_dot;

gradPhi = [2*x(1),0,0;...
             x(2),x(1),0;...
             x(3),0,x(1);...
             0,2*x(2),0;...
             0,x(3),x(2);...
             0,0,2*x(3);...
              2*x(1)*x(7)^2,0,0;...
              0,2*x(2)*x(8)^2,0;...
              0,0,2*x(3)*x(9)^2;...
              2*x(1)*x(4)^2,0,0;...
              0,2*x(2)*x(5)^2,0;...
              0,0,2*x(3)*x(6)^2]; 
          %size 12x3
Phi = [x(1)^2; x(1)*x(2); x(1)*x(3); x(2)^2; x(2)*x(3); x(3)^2; x(1)^2*x(7)^2; x(2)^2*x(8)^2; ...
    x(3)^2*x(9)^2; x(1)^2*x(4)^2; x(2)^2*x(5)^2; x(3)^2*x(6)^2];
V = W_vc'*Phi;    
J = [cos(eta(3)),-sin(eta(3)),0;sin(eta(3)),cos(eta(3)),0;0,0,1];

J_dot = [-sin(eta(3))*v(3), -cos(eta(3))*v(3), 0;
      cos(eta(3))*v(3), -sin(eta(3))*v(3), 0;
             0, 0, 0];
         

%%
v_d_dot = J_dot'*(eta_d_dot-beta_eta*z_eta)+J'*(eta_d_dot_dot-beta_eta*z_eta_dot);
delta_hjb = W_vc'*gradPhi*(v_dot-v_d_dot)+z_v'*z_v+u'*u;
omega = gradPhi*(v_dot-v_d_dot);    %size 12x1

W_vc_dot = -eta_c*GAMMA*omega/(1+nuy*(omega'*GAMMA*omega))*delta_hjb;
W_va_dot = -eta_a1/sqrt(1+omega'*omega)*gradPhi*(invM*invM')*gradPhi'*(W_va-W_vc)*delta_hjb...
-eta_a2*(W_va - W_vc);

tau_d = M*v_d_dot+C*v_d+D*v_d;

u = -1/2*invM'*gradPhi'*W_va;



tau = tau_d + u;
 end

== matlab function mpcfinal/Subsystem3/ADP and SV model3/Kinematic Control Law  ==
  data: eta_d input; v_d output; eta_d_dot input; eta input
function v_d = fcn(eta_d,eta_d_dot, eta)
beta_eta = 0.3;

J = [cos(eta(3)),-sin(eta(3)),0;sin(eta(3)),cos(eta(3)),0;0,0,1];
z_eta = eta - eta_d;
v_d = J'*(eta_d_dot-beta_eta*z_eta);
end

== matlab function mpcfinal/Subsystem3/ADP and SV model3/MATLAB Function ==
  data: x output; eta input; y output; phi output
function [x,y,phi] = fcn(eta)
x = eta(1);
y = eta(2);
phi = eta(3);

== matlab function mpcfinal/Subsystem3/ADP and SV model3/Surface Vessel  ==
  settings: updateMethod=DISCRETE
  data: t input; tau input; v_dot output; v input
function v_dot  = fcn(t, tau,v)
%%

M = [28.135,0,0;0,45.568,0;0,0,131.423];
C = [0,0,-45.568*v(2);0,0,28.135*v(1);-8.7165*v(2),-8.7165*v(1),0];
D = [100,0,0;0,200,0;0,0,150];
 
invM = inv(M);

%%
if (t < 15)
    flag = 1;
else 
    flag = 0;
end
noise = zeros(3,1);
% noise(1) = (50*sin(25*t) + 65*sin(45*(t-1)) + 45*sin(20*(t-0.5)) + 55*sin(35*(t-1.5)))*flag;
% noise(2) = (20*sin(25*t) + 10*sin(45*(t-1)) + 16*sin(20*(t-0.5)) + 20*sin(35*(t-1.5)))*flag;
% noise(3) = (9*sin(25*t) + 10*sin(45*(t-1)) + 14*sin(20*(t-0.5)) + 30*sin(35*(t-1.5)))*flag;

noise(1) = (10*sin(25*t) + 16*sin(45*(t-1)) + 15*sin(20*(t-0.5)) + 10*sin(35*(t-1.5)))*flag;
noise(2) = (50*sin(25*t) + 50*sin(45*(t-1)) + 40*sin(20*(t-0.5)) + 50*sin(35*(t-1.5)))*flag;
noise(3) = (40*sin(25*t) + 30*sin(45*(t-1)) + 45*sin(20*(t-0.5)) + 40*sin(35*(t-1.5)))*flag;

v_dot = -invM*C*v-invM*D*v+invM*(tau + noise);

== matlab function mpcfinal/Subsystem3/ADP and SV model3/v to eta_dot ==
  data: v input; eta_dot output; eta input
function eta_dot = fcn(v,eta)
J = [cos(eta(3)),-sin(eta(3)),0;sin(eta(3)),cos(eta(3)),0;0,0,1];
eta_dot = J*v;

== matlab function mpcfinal/Subsystem3/MATLAB Function ==
  data: t input; y output
function y = fcn(t)

y = [5+0.5*t+5*sin(0.05*t),10+0.5*t,0];
end

== matlab function mpcfinal/Subsystem/Transform to Theta dot ==
  data: u_d input; x_d_dot output; v_d input; r_d input; y_d_dot output; phi_d_dot output; psi input
function [x_d_dot,y_d_dot,phi_d_dot] = fcn(u_d,v_d,r_d,psi)
    x_d_dot = u_d*cos(psi) - v_d*sin(psi);
    y_d_dot = u_d*sin(psi) + v_d*cos(psi);
    phi_d_dot = r_d;

== matlab function mpcfinal/Subsystem3/Transform to Theta dot ==
  data: u_d input; x_d_dot output; v_d input; r_d input; y_d_dot output; phi_d_dot output; psi input
function [x_d_dot,y_d_dot,phi_d_dot] = fcn(u_d,v_d,r_d,psi)
    x_d_dot = u_d*cos(psi) - v_d*sin(psi);
    y_d_dot = u_d*sin(psi) + v_d*cos(psi);
    phi_d_dot = r_d;

== matlab function mpcfinal/Subsystem4/ADP and SV model3/ADP/Controller ==
  data: W_vc input; W_vc_dot output; W_va_dot output; tau_d output; W_va input; v_dot input; v_d input; v input; eta input; eta_dot input; eta_d input; eta_d_dot input; eta_d_dot_dot input; u input; u output; V output; tau output; z_eta output
 function [W_vc_dot, W_va_dot, tau_d, u, V, tau, z_eta] = fcn(W_vc, W_va, v_dot, v_d, v,...
    eta, eta_dot, eta_d, eta_d_dot, eta_d_dot_dot,u)
M = [28.135,0,0;0,45.568,0;0,0,131.423];
C = [0,0,-45.568*v(2);0,0,28.135*v(1);-8.7165*v(2),-8.7165*v(1),0];
D = [100,0,0;0,200,0;0,0,150];
invM = inv(M);
beta_eta = 0.3;
eta_c = 10;
eta_a1 = 10;
eta_a2 = 20;
nuy = 0.01;
GAMMA = 20; %%khong cap nhat
%%
z_eta = eta-eta_d;
z_v = v - v_d;
x = [z_v;z_eta;eta_d];
z_eta_dot = eta_dot - eta_d_dot;

gradPhi = [2*x(1),0,0;...
             x(2),x(1),0;...
             x(3),0,x(1);...
             0,2*x(2),0;...
             0,x(3),x(2);...
             0,0,2*x(3);...
              2*x(1)*x(7)^2,0,0;...
              0,2*x(2)*x(8)^2,0;...
              0,0,2*x(3)*x(9)^2;...
              2*x(1)*x(4)^2,0,0;...
              0,2*x(2)*x(5)^2,0;...
              0,0,2*x(3)*x(6)^2]; 
          %size 12x3
Phi = [x(1)^2; x(1)*x(2); x(1)*x(3); x(2)^2; x(2)*x(3); x(3)^2; x(1)^2*x(7)^2; x(2)^2*x(8)^2; ...
    x(3)^2*x(9)^2; x(1)^2*x(4)^2; x(2)^2*x(5)^2; x(3)^2*x(6)^2];
V = W_vc'*Phi;    
J = [cos(eta(3)),-sin(eta(3)),0;sin(eta(3)),cos(eta(3)),0;0,0,1];

J_dot = [-sin(eta(3))*v(3), -cos(eta(3))*v(3), 0;
      cos(eta(3))*v(3), -sin(eta(3))*v(3), 0;
             0, 0, 0];
         

%%
v_d_dot = J_dot'*(eta_d_dot-beta_eta*z_eta)+J'*(eta_d_dot_dot-beta_eta*z_eta_dot);
delta_hjb = W_vc'*gradPhi*(v_dot-v_d_dot)+z_v'*z_v+u'*u;
omega = gradPhi*(v_dot-v_d_dot);    %size 12x1

W_vc_dot = -eta_c*GAMMA*omega/(1+nuy*(omega'*GAMMA*omega))*delta_hjb;
W_va_dot = -eta_a1/sqrt(1+omega'*omega)*gradPhi*(invM*invM')*gradPhi'*(W_va-W_vc)*delta_hjb...
-eta_a2*(W_va - W_vc);

tau_d = M*v_d_dot+C*v_d+D*v_d;

u = -1/2*invM'*gradPhi'*W_va;



tau = tau_d + u;
 end

== matlab function mpcfinal/Subsystem1/ADP and SV model3/ADP/Controller ==
  data: W_vc input; W_vc_dot output; W_va_dot output; tau_d output; W_va input; v_dot input; v_d input; v input; eta input; eta_dot input; eta_d input; eta_d_dot input; eta_d_dot_dot input; u input; u output; V output; tau output; z_eta output
 function [W_vc_dot, W_va_dot, tau_d, u, V, tau, z_eta] = fcn(W_vc, W_va, v_dot, v_d, v,...
    eta, eta_dot, eta_d, eta_d_dot, eta_d_dot_dot,u)
M = [28.135,0,0;0,45.568,0;0,0,131.423];
C = [0,0,-45.568*v(2);0,0,28.135*v(1);-8.7165*v(2),-8.7165*v(1),0];
D = [100,0,0;0,200,0;0,0,150];
invM = inv(M);
beta_eta = 0.3;
eta_c = 10;
eta_a1 = 10;
eta_a2 = 20;
nuy = 0.01;
GAMMA = 20; %%khong cap nhat
%%
z_eta = eta-eta_d;
z_v = v - v_d;
x = [z_v;z_eta;eta_d];
z_eta_dot = eta_dot - eta_d_dot;

gradPhi = [2*x(1),0,0;...
             x(2),x(1),0;...
             x(3),0,x(1);...
             0,2*x(2),0;...
             0,x(3),x(2);...
             0,0,2*x(3);...
              2*x(1)*x(7)^2,0,0;...
              0,2*x(2)*x(8)^2,0;...
              0,0,2*x(3)*x(9)^2;...
              2*x(1)*x(4)^2,0,0;...
              0,2*x(2)*x(5)^2,0;...
              0,0,2*x(3)*x(6)^2]; 
          %size 12x3
Phi = [x(1)^2; x(1)*x(2); x(1)*x(3); x(2)^2; x(2)*x(3); x(3)^2; x(1)^2*x(7)^2; x(2)^2*x(8)^2; ...
    x(3)^2*x(9)^2; x(1)^2*x(4)^2; x(2)^2*x(5)^2; x(3)^2*x(6)^2];
V = W_vc'*Phi;    
J = [cos(eta(3)),-sin(eta(3)),0;sin(eta(3)),cos(eta(3)),0;0,0,1];

J_dot = [-sin(eta(3))*v(3), -cos(eta(3))*v(3), 0;
      cos(eta(3))*v(3), -sin(eta(3))*v(3), 0;
             0, 0, 0];
         

%%
v_d_dot = J_dot'*(eta_d_dot-beta_eta*z_eta)+J'*(eta_d_dot_dot-beta_eta*z_eta_dot);
delta_hjb = W_vc'*gradPhi*(v_dot-v_d_dot)+z_v'*z_v+u'*u;
omega = gradPhi*(v_dot-v_d_dot);    %size 12x1

W_vc_dot = -eta_c*GAMMA*omega/(1+nuy*(omega'*GAMMA*omega))*delta_hjb;
W_va_dot = -eta_a1/sqrt(1+omega'*omega)*gradPhi*(invM*invM')*gradPhi'*(W_va-W_vc)*delta_hjb...
-eta_a2*(W_va - W_vc);

tau_d = M*v_d_dot+C*v_d+D*v_d;

u = -1/2*invM'*gradPhi'*W_va;



tau = tau_d + u;
 end

== matlab function mpcfinal/Subsystem4/ADP and SV model3/Kinematic Control Law  ==
  data: eta_d input; v_d output; eta_d_dot input; eta input
function v_d = fcn(eta_d,eta_d_dot, eta)
beta_eta = 0.3;

J = [cos(eta(3)),-sin(eta(3)),0;sin(eta(3)),cos(eta(3)),0;0,0,1];
z_eta = eta - eta_d;
v_d = J'*(eta_d_dot-beta_eta*z_eta);
end

== matlab function mpcfinal/Subsystem4/ADP and SV model3/MATLAB Function ==
  data: x output; eta input; y output; phi output
function [x,y,phi] = fcn(eta)
x = eta(1);
y = eta(2);
phi = eta(3);

== matlab function mpcfinal/Subsystem4/ADP and SV model3/Surface Vessel  ==
  settings: updateMethod=DISCRETE
  data: t input; tau input; v_dot output; v input
function v_dot  = fcn(t, tau,v)
%%

M = [28.135,0,0;0,45.568,0;0,0,131.423];
C = [0,0,-45.568*v(2);0,0,28.135*v(1);-8.7165*v(2),-8.7165*v(1),0];
D = [100,0,0;0,200,0;0,0,150];
 
invM = inv(M);

%%
if (t < 15)
    flag = 1;
else 
    flag = 0;
end
noise = zeros(3,1);
% noise(1) = (50*sin(25*t) + 65*sin(45*(t-1)) + 45*sin(20*(t-0.5)) + 55*sin(35*(t-1.5)))*flag;
% noise(2) = (20*sin(25*t) + 10*sin(45*(t-1)) + 16*sin(20*(t-0.5)) + 20*sin(35*(t-1.5)))*flag;
% noise(3) = (9*sin(25*t) + 10*sin(45*(t-1)) + 14*sin(20*(t-0.5)) + 30*sin(35*(t-1.5)))*flag;

noise(1) = (10*sin(25*t) + 16*sin(45*(t-1)) + 15*sin(20*(t-0.5)) + 10*sin(35*(t-1.5)))*flag;
noise(2) = (50*sin(25*t) + 50*sin(45*(t-1)) + 40*sin(20*(t-0.5)) + 50*sin(35*(t-1.5)))*flag;
noise(3) = (40*sin(25*t) + 30*sin(45*(t-1)) + 45*sin(20*(t-0.5)) + 40*sin(35*(t-1.5)))*flag;

v_dot = -invM*C*v-invM*D*v+invM*(tau + noise);

== matlab function mpcfinal/Subsystem4/ADP and SV model3/v to eta_dot ==
  data: v input; eta_dot output; eta input
function eta_dot = fcn(v,eta)
J = [cos(eta(3)),-sin(eta(3)),0;sin(eta(3)),cos(eta(3)),0;0,0,1];
eta_dot = J*v;

== matlab function mpcfinal/Subsystem4/MATLAB Function ==
  data: t input; y output
function y = fcn(t)

y = [10+0.5*t+5*sin(0.05*t),15+0.5*t,0];
end

== matlab function mpcfinal/Subsystem4/Transform to Theta dot ==
  data: u_d input; x_d_dot output; v_d input; r_d input; y_d_dot output; phi_d_dot output; psi input
function [x_d_dot,y_d_dot,phi_d_dot] = fcn(u_d,v_d,r_d,psi)
    x_d_dot = u_d*cos(psi) - v_d*sin(psi);
    y_d_dot = u_d*sin(psi) + v_d*cos(psi);
    phi_d_dot = r_d;

== matlab function mpcfinal/Variable exchange ==
  data: x1 input; xy output; y1 input; x2 input; y2 input; x3 input; y3 input; x4 input; y4 input; x5 input; y5 input; x output; y output
function [xy,x,y] = fcn(x1,y1,x2,y2,x3,y3,x4,y4,x5,y5)

xy = [x1;y1;x2;y2;x3;y3;x4;y4;x5;y5];
x = [x1;x2;x3;x4;x5];
y = [y1;y2;y3;y4;y5];

== matlab function mpcfinal/Subsystem/ADP and SV model3/ADP/Controller ==
  data: W_vc input; W_vc_dot output; W_va_dot output; tau_d output; W_va input; v_dot input; v_d input; v input; eta input; eta_dot input; eta_d input; eta_d_dot input; eta_d_dot_dot input; u input; u output; V output; tau output; z_eta output
 function [W_vc_dot, W_va_dot, tau_d, u, V, tau, z_eta] = fcn(W_vc, W_va, v_dot, v_d, v,...
    eta, eta_dot, eta_d, eta_d_dot, eta_d_dot_dot,u)
M = [28.135,0,0;0,45.568,0;0,0,131.423];
C = [0,0,-45.568*v(2);0,0,28.135*v(1);-8.7165*v(2),-8.7165*v(1),0];
D = [100,0,0;0,200,0;0,0,150];
invM = inv(M);
beta_eta = 0.3;
eta_c = 10;
eta_a1 = 10;
eta_a2 = 20;
nuy = 0.01;
GAMMA = 20; %%khong cap nhat
%%
z_eta = eta-eta_d;
z_v = v - v_d;
x = [z_v;z_eta;eta_d];
z_eta_dot = eta_dot - eta_d_dot;

gradPhi = [2*x(1),0,0;...
             x(2),x(1),0;...
             x(3),0,x(1);...
             0,2*x(2),0;...
             0,x(3),x(2);...
             0,0,2*x(3);...
              2*x(1)*x(7)^2,0,0;...
              0,2*x(2)*x(8)^2,0;...
              0,0,2*x(3)*x(9)^2;...
              2*x(1)*x(4)^2,0,0;...
              0,2*x(2)*x(5)^2,0;...
              0,0,2*x(3)*x(6)^2]; 
          %size 12x3
Phi = [x(1)^2; x(1)*x(2); x(1)*x(3); x(2)^2; x(2)*x(3); x(3)^2; x(1)^2*x(7)^2; x(2)^2*x(8)^2; ...
    x(3)^2*x(9)^2; x(1)^2*x(4)^2; x(2)^2*x(5)^2; x(3)^2*x(6)^2];
V = W_vc'*Phi;    
J = [cos(eta(3)),-sin(eta(3)),0;sin(eta(3)),cos(eta(3)),0;0,0,1];

J_dot = [-sin(eta(3))*v(3), -cos(eta(3))*v(3), 0;
      cos(eta(3))*v(3), -sin(eta(3))*v(3), 0;
             0, 0, 0];
         

%%
v_d_dot = J_dot'*(eta_d_dot-beta_eta*z_eta)+J'*(eta_d_dot_dot-beta_eta*z_eta_dot);
delta_hjb = W_vc'*gradPhi*(v_dot-v_d_dot)+z_v'*z_v+u'*u;
omega = gradPhi*(v_dot-v_d_dot);    %size 12x1

W_vc_dot = -eta_c*GAMMA*omega/(1+nuy*(omega'*GAMMA*omega))*delta_hjb;
W_va_dot = -eta_a1/sqrt(1+omega'*omega)*gradPhi*(invM*invM')*gradPhi'*(W_va-W_vc)*delta_hjb...
-eta_a2*(W_va - W_vc);

tau_d = M*v_d_dot+C*v_d+D*v_d;

u = -1/2*invM'*gradPhi'*W_va;



tau = tau_d + u;
 end

== matlab function mpcfinal/Subsystem/ADP and SV model3/Kinematic Control Law  ==
  data: eta_d input; v_d output; eta_d_dot input; eta input
function v_d = fcn(eta_d,eta_d_dot, eta)
beta_eta = 0.3;

J = [cos(eta(3)),-sin(eta(3)),0;sin(eta(3)),cos(eta(3)),0;0,0,1];
z_eta = eta - eta_d;
v_d = J'*(eta_d_dot-beta_eta*z_eta);
end

== matlab function mpcfinal/Subsystem/ADP and SV model3/MATLAB Function ==
  data: x output; eta input; y output; phi output
function [x,y,phi] = fcn(eta)
x = eta(1);
y = eta(2);
phi = eta(3);

== matlab function mpcfinal/Subsystem/ADP and SV model3/Surface Vessel  ==
  settings: updateMethod=DISCRETE
  data: t input; tau input; v_dot output; v input
function v_dot  = fcn(t, tau,v)
%%

M = [28.135,0,0;0,45.568,0;0,0,131.423];
C = [0,0,-45.568*v(2);0,0,28.135*v(1);-8.7165*v(2),-8.7165*v(1),0];
D = [100,0,0;0,200,0;0,0,150];
 
invM = inv(M);

%%
if (t < 15)
    flag = 1;
else 
    flag = 0;
end
noise = zeros(3,1);
% noise(1) = (50*sin(25*t) + 65*sin(45*(t-1)) + 45*sin(20*(t-0.5)) + 55*sin(35*(t-1.5)))*flag;
% noise(2) = (20*sin(25*t) + 10*sin(45*(t-1)) + 16*sin(20*(t-0.5)) + 20*sin(35*(t-1.5)))*flag;
% noise(3) = (9*sin(25*t) + 10*sin(45*(t-1)) + 14*sin(20*(t-0.5)) + 30*sin(35*(t-1.5)))*flag;

noise(1) = (10*sin(25*t) + 16*sin(45*(t-1)) + 15*sin(20*(t-0.5)) + 10*sin(35*(t-1.5)))*flag;
noise(2) = (50*sin(25*t) + 50*sin(45*(t-1)) + 40*sin(20*(t-0.5)) + 50*sin(35*(t-1.5)))*flag;
noise(3) = (40*sin(25*t) + 30*sin(45*(t-1)) + 45*sin(20*(t-0.5)) + 40*sin(35*(t-1.5)))*flag;

v_dot = -invM*C*v-invM*D*v+invM*(tau + noise);

== matlab function mpcfinal/Subsystem/ADP and SV model3/v to eta_dot ==
  data: v input; eta_dot output; eta input
function eta_dot = fcn(v,eta)
J = [cos(eta(3)),-sin(eta(3)),0;sin(eta(3)),cos(eta(3)),0;0,0,1];
eta_dot = J*v;

== matlab function mpcfinal/Subsystem/MATLAB Function ==
  data: t input; y output
function y = fcn(t)

y = [10+0.5*t+5*sin(0.05*t),10+0.5*t,0];
end

== matlab function mpcfinal/Subsystem1/ADP and SV model3/Kinematic Control Law  ==
  data: eta_d input; v_d output; eta_d_dot input; eta input
function v_d = fcn(eta_d,eta_d_dot, eta)
beta_eta = 0.3;

J = [cos(eta(3)),-sin(eta(3)),0;sin(eta(3)),cos(eta(3)),0;0,0,1];
z_eta = eta - eta_d;
v_d = J'*(eta_d_dot-beta_eta*z_eta);
end

== matlab function mpcfinal/Subsystem1/ADP and SV model3/MATLAB Function ==
  data: x output; eta input; y output; phi output
function [x,y,phi] = fcn(eta)
x = eta(1);
y = eta(2);
phi = eta(3);

== matlab function mpcfinal/Subsystem1/ADP and SV model3/Surface Vessel  ==
  settings: updateMethod=DISCRETE
  data: t input; tau input; v_dot output; v input
function v_dot  = fcn(t, tau,v)
%%

M = [28.135,0,0;0,45.568,0;0,0,131.423];
C = [0,0,-45.568*v(2);0,0,28.135*v(1);-8.7165*v(2),-8.7165*v(1),0];
D = [100,0,0;0,200,0;0,0,150];
 
invM = inv(M);

%%
if (t < 15)
    flag = 1;
else 
    flag = 0;
end
noise = zeros(3,1);
% noise(1) = (50*sin(25*t) + 65*sin(45*(t-1)) + 45*sin(20*(t-0.5)) + 55*sin(35*(t-1.5)))*flag;
% noise(2) = (20*sin(25*t) + 10*sin(45*(t-1)) + 16*sin(20*(t-0.5)) + 20*sin(35*(t-1.5)))*flag;
% noise(3) = (9*sin(25*t) + 10*sin(45*(t-1)) + 14*sin(20*(t-0.5)) + 30*sin(35*(t-1.5)))*flag;

noise(1) = (10*sin(25*t) + 16*sin(45*(t-1)) + 15*sin(20*(t-0.5)) + 10*sin(35*(t-1.5)))*flag;
noise(2) = (50*sin(25*t) + 50*sin(45*(t-1)) + 40*sin(20*(t-0.5)) + 50*sin(35*(t-1.5)))*flag;
noise(3) = (40*sin(25*t) + 30*sin(45*(t-1)) + 45*sin(20*(t-0.5)) + 40*sin(35*(t-1.5)))*flag;

v_dot = -invM*C*v-invM*D*v+invM*(tau + noise);

== matlab function mpcfinal/Subsystem1/ADP and SV model3/v to eta_dot ==
  data: v input; eta_dot output; eta input
function eta_dot = fcn(v,eta)
J = [cos(eta(3)),-sin(eta(3)),0;sin(eta(3)),cos(eta(3)),0;0,0,1];
eta_dot = J*v;

== matlab function mpcfinal/Subsystem1/MATLAB Function ==
  data: t input; y output
function y = fcn(t)

y = [15+0.5*t+5*sin(0.05*t),10+0.5*t,0];
end
